simulink model "CompleteModelSimulink"  (R2024a)
settings: Solver=ode45  StartTime=0.0  StopTime=endtime  RelTol=1e-3
values from neighbouring files (symbols this model uses):
  D = 0.069    [CompleteModel.m]
  D_H = 2    [PID_Current.m]    (also in PID_NoCurrent.m = 1)
  D_X = 2    [PID_Current.m]    (also in PID_NoCurrent.m = 1.05)
  D_Y = 2    [PID_Current.m]    (also in PID_NoCurrent.m = 0.8)
  DC =     [DC.mat]
  I_H = 0.1    [PID_Current.m]    (also in PID_NoCurrent.m = 0.01)
  I_X = 0.1    [PID_Current.m]    (also in PID_NoCurrent.m = 0.001)
  I_Y = 0.2    [PID_Current.m]    (also in PID_NoCurrent.m = 0.01)
  InitialPos = [0;0;0]    [CompleteModel.m]
  M_matrix = [2.5 0 0; 0 2.50 0; 0 0 1]    [CompleteModel.m]
  P_H = 2    [PID_Current.m]    (also in PID_NoCurrent.m = 1)
  P_X = 2    [PID_Current.m]    (also in PID_NoCurrent.m = 0.75)
  P_Y = 2    [PID_Current.m]    (also in PID_NoCurrent.m = 1.3)
  Ref = [1;0;0]    [CompleteModel.m]
  SpeedFactor = 0.07    [CompleteModel.m]
  SR =     [SR.mat]
  T_matrix = [0 1 0; 1 0 1; 0.35 -0.065 -0.35]    [CompleteModel.m]
  TauE = [-0.15;0;0]    [CompleteModel.m]
libraries: slpidlib x8
(part 1 of 2)
settings Model: Creator=31620  LastModifiedBy=31620
settings SolverCC: AlgebraicLoopSolver=TrustRegion
settings DebuggingCC: UnconnectedInputMsg=warning  UnconnectedOutputMsg=warning  UnconnectedLineMsg=warning
settings ModelReferenceCC: EnableRefExpFcnMdlSchedulingChecks=on
settings RTWCC: GPUComputeCapability=3.5

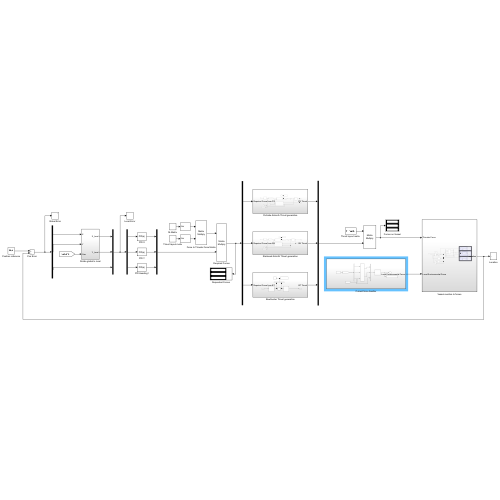
[thumbnail: Simulink's stored preview of the top-level diagram]
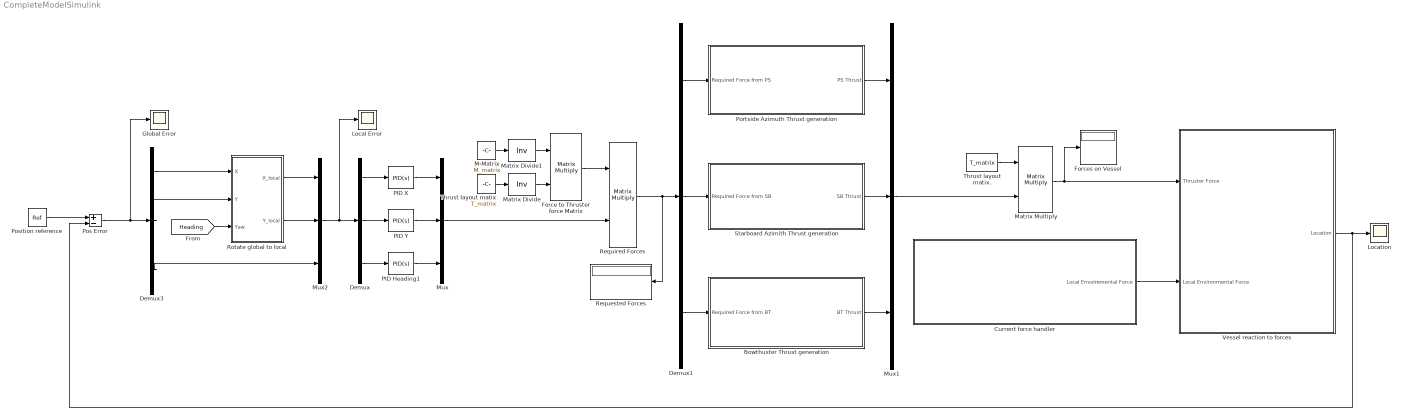
== system CompleteModelSimulink ==
  Bowthuster Thrust generation : Subsystem
  Current force handler : Subsystem
  Demux : Demux  Outputs=3
  Demux1 : Demux  Outputs=3
  Demux3 : Demux  Outputs=3
  Force to Thruster force Matrix : Product  Multiplication=Matrix(*)
  Forces on Vessel : Display
  Global Error : Scope
  Local Error : Scope
  Location : Scope
  M-Matrix : Constant  Value=M_matrix
  Matrix Divide : Product  Inputs=/  Multiplication=Matrix(*)
  Matrix Divide1 : Product  Inputs=/  Multiplication=Matrix(*)
  Matrix Multiply : Product  Multiplication=Matrix(*)
  Mux : Mux  Inputs=3
  Mux1 : Mux  Inputs=3
  Mux2 : Mux  Inputs=3
  PID Heading1 : slpidlib/PID Controller  Controller=PID  Form=Parallel  TimeDomain=Continuous-time  UseExternalTs=off  SampleTime=-1  IntegratorMethod=Forward Euler  FilterMethod=Forward Euler  ControllerParametersSource=internal  P=P_H  I=I_H  UseKiTs=off  D=D_H  UseExternalDerivativeSource=off  N=10000  UseFilter=on  TunerSelectOption=Transfer Function Based (PID Tuner App)  InitialConditionSource=internal  InitialConditionForIntegrator=0  InitialConditionForFilter=0  DifferentiatorICPrevScaledInput=0  ExternalReset=none  TrackingMode=off  Kt=1  LimitOutput=off  SatLimitsSource=internal  UpperSaturationLimit=inf  LowerSaturationLimit=-inf  LinearizeAsGain=on  AntiWindupMode=none  Kb=1  LimitIntegrator=off  UpperIntegratorSaturationLimit=inf  LowerIntegratorSaturationLimit=-inf  POutMin=[]  POutMax=[]  IOutMin=[]  IOutMax=[]  DOutMin=[]  DOutMax=[]  NOutMin=[]  NOutMax=[]  SumOutMin=[]  SumOutMax=[]  SaturationOutMin=[]  SaturationOutMax=[]  PParamMin=[]  PParamMax=[]  IParamMin=[]  IParamMax=[]  DParamMin=[]  DParamMax=[]  NParamMin=[]  NParamMax=[]  KbParamMin=[]  KbParamMax=[]  KtParamMin=[]  KtParamMax=[]  KbOutMin=[]  KbOutMax=[]  KtOutMin=[]  KtOutMax=[]  IntegratorOutMin=[]  IntegratorOutMax=[]  FilterOutMin=[]  FilterOutMax=[]  SumI1OutMin=[]  SumI1OutMax=[]  SumI2OutMin=[]  SumI2OutMax=[]  SumI3OutMin=[]  SumI3OutMax=[]  SumI4OutMin=[]  SumI4OutMax=[]  SumDOutMin=[]  SumDOutMax=[]  DifferentiatorOutMin=[]  DifferentiatorOutMax=[]  FilterDiffOutCoefMin=[]  FilterDiffOutCoefMax=[]  ReciprocalOutMin=[]  ReciprocalOutMax=[]  SumDenOutMin=[]  SumDenOutMax=[]  SumNumOutMin=[]  SumNumOutMax=[]  DivideOutMin=[]  DivideOutMax=[]  UdiffTsProdOutMin=[]  UdiffTsProdOutMax=[]  NTsProdOutMin=[]  NTsProdOutMax=[]  UintegralTsProdOutMin=[]  UintegralTsProdOutMax=[]  UngainTsProdOutMin=[]  UngainTsProdOutMax=[]  ClampingZeroOutDataTypeStr=Inherit: Inherit via back propagation  ClampingZeroOutMin=[]  ClampingZeroOutMax=[]  FilterDenConstantOutDataTypeStr=Inherit: Inherit via back propagation  FilterDenConstantOutMin=[]  FilterDenConstantOutMax=[]  PCopyOutDataTypeStr=Inherit: Inherit via back propagation  PCopyOutMin=[]  PCopyOutMax=[]  NCopyOutDataTypeStr=Inherit: Inherit via back propagation  NCopyOutMin=[]  NCopyOutMax=[]  IntegratorContinuousStateAttributes=''  IntegratorStateMustResolveToSignalObject=off  IntegratorRTWStateStorageClass=Auto  FilterContinuousStateAttributes=''  FilterStateMustResolveToSignalObject=off  FilterRTWStateStorageClass=Auto  ParallelPVariant=InternalParameters  IdealPVariant=Disabled  IVariant=InternalParameters  DVariant=InternalParameters  IntegratorVariant=Continuous  SatVariant=Disabled  AWVariant=Passthrough  PCopyVariant=Disabled  TRVariant=Disabled  FdbkBlocksVariant=Forward  IdealPFdbkVariant=Disabled  SatFdbkVariant=Disabled  DerivativeFilterVariant=ContFilter  NVariant=InternalParameters  NCopyVariant=Disabled  FilterICVariant=InternalICsFilter  IntegratorICVariant=InternalICs  ExternalResetVariant=Disabled  TRSumVariant=Passthrough  SumFdbkVariant=Disabled  SumVariant=Sum_PID  TsampFilterVariant=InternalTs  TsampNgainVariant=Passthrough  TsampIntegralVariant=Disabled_SignalSpec  ExternalSaturationOutDataTypeStr=Inherit: Same as second input  DerivativeSourceVariant=ErrorSignal
  PID X : slpidlib/PID Controller  Controller=PID  Form=Parallel  TimeDomain=Continuous-time  UseExternalTs=off  SampleTime=-1  IntegratorMethod=Forward Euler  FilterMethod=Forward Euler  ControllerParametersSource=internal  P=P_X  I=I_X  UseKiTs=off  D=D_X  UseExternalDerivativeSource=off  N=10000  UseFilter=on  TunerSelectOption=Transfer Function Based (PID Tuner App)  InitialConditionSource=internal  InitialConditionForIntegrator=0  InitialConditionForFilter=0  DifferentiatorICPrevScaledInput=0  ExternalReset=none  TrackingMode=off  Kt=1  LimitOutput=off  SatLimitsSource=internal  UpperSaturationLimit=inf  LowerSaturationLimit=-inf  LinearizeAsGain=on  AntiWindupMode=none  Kb=1  LimitIntegrator=off  UpperIntegratorSaturationLimit=inf  LowerIntegratorSaturationLimit=-inf  POutMin=[]  POutMax=[]  IOutMin=[]  IOutMax=[]  DOutMin=[]  DOutMax=[]  NOutMin=[]  NOutMax=[]  SumOutMin=[]  SumOutMax=[]  SaturationOutMin=[]  SaturationOutMax=[]  PParamMin=[]  PParamMax=[]  IParamMin=[]  IParamMax=[]  DParamMin=[]  DParamMax=[]  NParamMin=[]  NParamMax=[]  KbParamMin=[]  KbParamMax=[]  KtParamMin=[]  KtParamMax=[]  KbOutMin=[]  KbOutMax=[]  KtOutMin=[]  KtOutMax=[]  IntegratorOutMin=[]  IntegratorOutMax=[]  FilterOutMin=[]  FilterOutMax=[]  SumI1OutMin=[]  SumI1OutMax=[]  SumI2OutMin=[]  SumI2OutMax=[]  SumI3OutMin=[]  SumI3OutMax=[]  SumI4OutMin=[]  SumI4OutMax=[]  SumDOutMin=[]  SumDOutMax=[]  DifferentiatorOutMin=[]  DifferentiatorOutMax=[]  FilterDiffOutCoefMin=[]  FilterDiffOutCoefMax=[]  ReciprocalOutMin=[]  ReciprocalOutMax=[]  SumDenOutMin=[]  SumDenOutMax=[]  SumNumOutMin=[]  SumNumOutMax=[]  DivideOutMin=[]  DivideOutMax=[]  UdiffTsProdOutMin=[]  UdiffTsProdOutMax=[]  NTsProdOutMin=[]  NTsProdOutMax=[]  UintegralTsProdOutMin=[]  UintegralTsProdOutMax=[]  UngainTsProdOutMin=[]  UngainTsProdOutMax=[]  ClampingZeroOutDataTypeStr=Inherit: Inherit via back propagation  ClampingZeroOutMin=[]  ClampingZeroOutMax=[]  FilterDenConstantOutDataTypeStr=Inherit: Inherit via back propagation  FilterDenConstantOutMin=[]  FilterDenConstantOutMax=[]  PCopyOutDataTypeStr=Inherit: Inherit via back propagation  PCopyOutMin=[]  PCopyOutMax=[]  NCopyOutDataTypeStr=Inherit: Inherit via back propagation  NCopyOutMin=[]  NCopyOutMax=[]  IntegratorContinuousStateAttributes=''  IntegratorStateMustResolveToSignalObject=off  IntegratorRTWStateStorageClass=Auto  FilterContinuousStateAttributes=''  FilterStateMustResolveToSignalObject=off  FilterRTWStateStorageClass=Auto  ParallelPVariant=InternalParameters  IdealPVariant=Disabled  IVariant=InternalParameters  DVariant=InternalParameters  IntegratorVariant=Continuous  SatVariant=Disabled  AWVariant=Passthrough  PCopyVariant=Disabled  TRVariant=Disabled  FdbkBlocksVariant=Forward  IdealPFdbkVariant=Disabled  SatFdbkVariant=Disabled  DerivativeFilterVariant=ContFilter  NVariant=InternalParameters  NCopyVariant=Disabled  FilterICVariant=InternalICsFilter  IntegratorICVariant=InternalICs  ExternalResetVariant=Disabled  TRSumVariant=Passthrough  SumFdbkVariant=Disabled  SumVariant=Sum_PID  TsampFilterVariant=InternalTs  TsampNgainVariant=Passthrough  TsampIntegralVariant=Disabled_SignalSpec  ExternalSaturationOutDataTypeStr=Inherit: Same as second input  DerivativeSourceVariant=ErrorSignal
  PID Y : slpidlib/PID Controller  Controller=PID  Form=Parallel  TimeDomain=Continuous-time  UseExternalTs=off  SampleTime=-1  IntegratorMethod=Forward Euler  FilterMethod=Forward Euler  ControllerParametersSource=internal  P=P_Y  I=I_Y  UseKiTs=off  D=D_Y  UseExternalDerivativeSource=off  N=10000  UseFilter=on  TunerSelectOption=Transfer Function Based (PID Tuner App)  InitialConditionSource=internal  InitialConditionForIntegrator=0  InitialConditionForFilter=0  DifferentiatorICPrevScaledInput=0  ExternalReset=none  TrackingMode=off  Kt=1  LimitOutput=off  SatLimitsSource=internal  UpperSaturationLimit=inf  LowerSaturationLimit=-inf  LinearizeAsGain=on  AntiWindupMode=none  Kb=1  LimitIntegrator=off  UpperIntegratorSaturationLimit=inf  LowerIntegratorSaturationLimit=-inf  POutMin=[]  POutMax=[]  IOutMin=[]  IOutMax=[]  DOutMin=[]  DOutMax=[]  NOutMin=[]  NOutMax=[]  SumOutMin=[]  SumOutMax=[]  SaturationOutMin=[]  SaturationOutMax=[]  PParamMin=[]  PParamMax=[]  IParamMin=[]  IParamMax=[]  DParamMin=[]  DParamMax=[]  NParamMin=[]  NParamMax=[]  KbParamMin=[]  KbParamMax=[]  KtParamMin=[]  KtParamMax=[]  KbOutMin=[]  KbOutMax=[]  KtOutMin=[]  KtOutMax=[]  IntegratorOutMin=[]  IntegratorOutMax=[]  FilterOutMin=[]  FilterOutMax=[]  SumI1OutMin=[]  SumI1OutMax=[]  SumI2OutMin=[]  SumI2OutMax=[]  SumI3OutMin=[]  SumI3OutMax=[]  SumI4OutMin=[]  SumI4OutMax=[]  SumDOutMin=[]  SumDOutMax=[]  DifferentiatorOutMin=[]  DifferentiatorOutMax=[]  FilterDiffOutCoefMin=[]  FilterDiffOutCoefMax=[]  ReciprocalOutMin=[]  ReciprocalOutMax=[]  SumDenOutMin=[]  SumDenOutMax=[]  SumNumOutMin=[]  SumNumOutMax=[]  DivideOutMin=[]  DivideOutMax=[]  UdiffTsProdOutMin=[]  UdiffTsProdOutMax=[]  NTsProdOutMin=[]  NTsProdOutMax=[]  UintegralTsProdOutMin=[]  UintegralTsProdOutMax=[]  UngainTsProdOutMin=[]  UngainTsProdOutMax=[]  ClampingZeroOutDataTypeStr=Inherit: Inherit via back propagation  ClampingZeroOutMin=[]  ClampingZeroOutMax=[]  FilterDenConstantOutDataTypeStr=Inherit: Inherit via back propagation  FilterDenConstantOutMin=[]  FilterDenConstantOutMax=[]  PCopyOutDataTypeStr=Inherit: Inherit via back propagation  PCopyOutMin=[]  PCopyOutMax=[]  NCopyOutDataTypeStr=Inherit: Inherit via back propagation  NCopyOutMin=[]  NCopyOutMax=[]  IntegratorContinuousStateAttributes=''  IntegratorStateMustResolveToSignalObject=off  IntegratorRTWStateStorageClass=Auto  FilterContinuousStateAttributes=''  FilterStateMustResolveToSignalObject=off  FilterRTWStateStorageClass=Auto  ParallelPVariant=InternalParameters  IdealPVariant=Disabled  IVariant=InternalParameters  DVariant=InternalParameters  IntegratorVariant=Continuous  SatVariant=Disabled  AWVariant=Passthrough  PCopyVariant=Disabled  TRVariant=Disabled  FdbkBlocksVariant=Forward  IdealPFdbkVariant=Disabled  SatFdbkVariant=Disabled  DerivativeFilterVariant=ContFilter  NVariant=InternalParameters  NCopyVariant=Disabled  FilterICVariant=InternalICsFilter  IntegratorICVariant=InternalICs  ExternalResetVariant=Disabled  TRSumVariant=Passthrough  SumFdbkVariant=Disabled  SumVariant=Sum_PID  TsampFilterVariant=InternalTs  TsampNgainVariant=Passthrough  TsampIntegralVariant=Disabled_SignalSpec  ExternalSaturationOutDataTypeStr=Inherit: Same as second input  DerivativeSourceVariant=ErrorSignal
  Portside Azimuth Thrust generation : Subsystem
  Pos Error : Sum  Inputs=+-
  Position reference : Constant  Value=Ref
  Requested Forces : Display
  Required Forces : Product  Multiplication=Matrix(*)
  "Rotate global to local " : Subsystem
  Starboard Azimith Thrust generation : Subsystem
  Thrust layout matix : Constant  Value=T_matrix
  Thrust layout matix. : Constant  Value=T_matrix
  Vessel reaction to forces : Subsystem
  wires:
  Position reference/1 -> Pos Error/1
  Demux/1 -> PID X/1
  Demux/2 -> PID Y/1
  Demux/3 -> PID Heading1/1
  Thrust layout matix/1 -> Matrix Divide/1
  M-Matrix/1 -> Matrix Divide1/1
  Matrix Divide/1 -> Force to Thruster force Matrix/2
  Force to Thruster force Matrix/1 -> Required Forces/1
  Required Forces/1 -> Demux1/1, Requested Forces/1
  Mux1/1 -> Matrix Multiply/2
  Matrix Multiply/1 -> Vessel reaction to forces/1(Thruster Force), Forces on Vessel/1
  Thrust layout matix./1 -> Matrix Multiply/1
  Vessel reaction to forces/1(Location) -> Pos Error/2, Location/1
  Mux/1 -> Required Forces/2
  [Heading] -> "Rotate global to local "/3(Yaw)
  "Rotate global to local "/1(X_local) -> Mux2/1
  "Rotate global to local "/2(Y_local) -> Mux2/2
  Mux2/1 -> Demux/1, Local Error/1
  Demux3/1 -> "Rotate global to local "/1(X)
  Demux3/2 -> "Rotate global to local "/2(Y)
  Pos Error/1 -> Global Error/1, Demux3/1
  Demux3/3 -> Mux2/3
  Matrix Divide1/1 -> Force to Thruster force Matrix/1
  PID Heading1/1 -> Mux/3
  PID Y/1 -> Mux/2
  PID X/1 -> Mux/1
  Demux1/1 -> Portside Azimuth Thrust generation/1(Required Force from PS)
  Portside Azimuth Thrust generation/1(PS Thrust) -> Mux1/1
  Demux1/2 -> Starboard Azimith Thrust generation/1(Required Force from SB)
  Starboard Azimith Thrust generation/1(SB Thrust) -> Mux1/2
  Demux1/3 -> Bowthuster Thrust generation/1(Required Force from BT)
  Bowthuster Thrust generation/1(BT Thrust) -> Mux1/3
  Current force handler/1(Local Envoiremental Force) -> Vessel reaction to forces/2(Local Environmental Force)

== system CompleteModelSimulink/Bowthuster Thrust generation ==
  Required Force from BT : Inport
  "Bow Thruster gain " : Scope
  Force to gain BT : Lookup_n-D  NumberOfTableDimensions=1  BreakpointsForDimension1=[-1.6375;-1.217;-1.0575;-0.92213;-0.78679;-0.47744;-0.16327;-0.005908;0;0.001074;0.059076;0.20892;0.54243;0.73093;1.0016;1.2385;1.3786;1.5526;1.8378]  Table=[-0.64591;-0.54475;-0.49416;-0.44358;-0.39377;-0.2965;-0.19611;-0.098054;0;0.10272;0.20545;0.25214;0.35254;0.40311;0.44825;0.50117;0.55331;0.59922;0.65214]  InternalRulePriority=Speed  RndMeth=Simplest
  Gain to Force BT : Lookup_n-D  NumberOfTableDimensions=1  BreakpointsForDimension1="[-0.645910 -0.544750 -0.49416 -0.443580 -0.39377 -0.2965 -0.19611 -0.098054  0.102720 0.20545 0.25214 0.35254 0.40311 0.448250 0.50117 0.55331 0.59922 0.65214]"  Table="[-1.6375 -1.217 -1.0575 -0.92213 -0.786790 -0.47744 -0.16327 -0.005908  0.001074 0.059076 0.20892 0.542430 0.73093 1.0016 1.2385 1.3786 1.5526 1.8378]"  InternalRulePriority=Speed  RndMeth=Simplest
  Mux6 : Mux  Inputs=2
  Saturation : Saturate  UpperLimit=0.6  LowerLimit=-0.6  ZeroCross=off
  To Workspace : ToWorkspace  VariableName=BowThruster  SaveFormat=Timeseries  SampleTime=-1
  BT Thrust : Outport
  wires:
  Required Force from BT/1 -> Force to gain BT/1
  Gain to Force BT/1 -> BT Thrust/1
  Mux6/1 -> To Workspace/1, "Bow Thruster gain "/1
  Saturation/1 -> Gain to Force BT/1, Mux6/2
  Force to gain BT/1 -> Saturation/1, Mux6/1

== system CompleteModelSimulink/Current force handler ==
  Current Forces : Subsystem
  Demux2 : Demux  Outputs=3
  Envoiremental Force : Constant  Value=TauE
  Gain : Gain  Gain=SpeedFactor
  Mux3 : Mux  Inputs=3
  Rotate global to local : Subsystem
  To Workspace : ToWorkspace  VariableName=LocalEnvoirmentalForce  SaveFormat=Timeseries  SampleTime=-1
  Local Envoiremental Force : Outport
  wires:
  Demux2/2 -> Rotate global to local/2(Y)
  [Heading] -> Rotate global to local/3(Yaw)
  Rotate global to local/2(Y_local) -> Mux3/2
  Demux2/1 -> Rotate global to local/1(X)
  Envoiremental Force/1 -> Gain/1
  Demux2/3 -> Mux3/3
  Gain/1 -> Demux2/1
  Rotate global to local/1(X_local) -> Mux3/1
  Mux3/1 -> Current Forces/1(Snelheid)
  Current Forces/1(D) -> To Workspace/1, Local Envoiremental Force/1

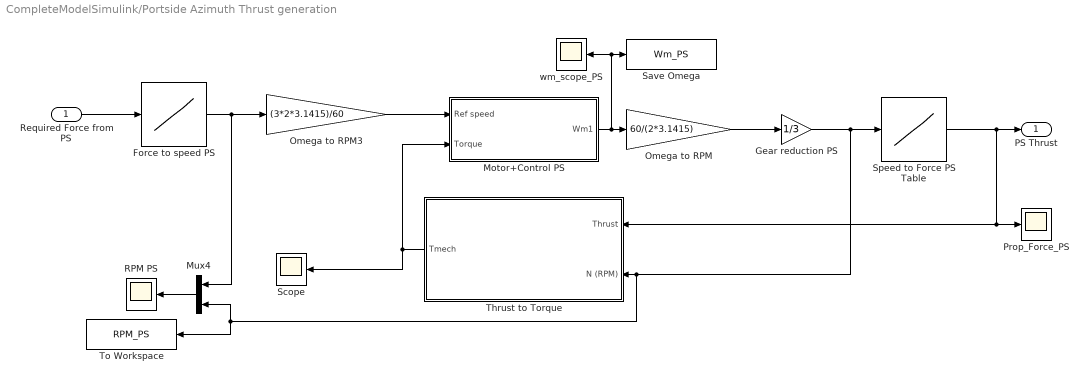
== system CompleteModelSimulink/Portside Azimuth Thrust generation ==
  Required Force from PS : Inport
  Force to speed PS : Lookup_n-D  NumberOfTableDimensions=1  BreakpointsForDimension1=[-2.338 -1.257 -1.059 -0.714 -0.499 -0.329 -0.159 -0.046 0 0.1011 0.2369 0.5481 0.882 1.4196 2.0251 2.789]  BreakpointsForDimension1DataTypeStr=Inherit: Inherit from 'Breakpoint data'  Table=[-998 -801.4 -762.5 -634.8 -563.7 -483.7 -397.1 -339.3 0 299.33 401.52 499.26 620.33 740.28 863.57 1000.2]  TableDataTypeStr=Inherit: Inherit from 'Table data'  RndMeth=Simplest
  Gear reduction PS : Gain  Gain=1/3
  Motor+Control PS : Subsystem
  Mux4 : Mux  Inputs=2
  Omega to RPM : Gain  Gain=60/(2*3.1415)
  Omega to RPM3 : Gain  Gain=(3*2*3.1415)/60
  Prop_Force_PS : Scope
  RPM PS : Scope
  Save Omega : ToWorkspace  VariableName=Wm_PS  SaveFormat=Timeseries  SampleTime=-1
  Scope : Scope
  Speed to Force PS Table : Lookup_n-D  NumberOfTableDimensions=1  BreakpointsForDimension1=[-998 -801.4 -762.5 -634.8 -563.7 -483.7 -397.1 -339.3 0 299.33 401.52 499.26 620.33 740.28 863.57 1000.2]  Table=[-2.338 -1.257 -1.059 -0.714 -0.499 -0.329 -0.159 -0.046 0 0.1011 0.2369 0.5481 0.882 1.4196 2.0251 2.789]  InternalRulePriority=Speed  RndMeth=Simplest
  Thrust to Torque : Subsystem
  To Workspace : ToWorkspace  VariableName=RPM_PS  SaveFormat=Timeseries  SampleTime=-1
  wm_scope_PS : Scope
  PS Thrust : Outport
  wires:
  Mux4/1 -> RPM PS/1
  Speed to Force PS Table/1 -> Thrust to Torque/1(Thrust), Prop_Force_PS/1, PS Thrust/1
  Force to speed PS/1 -> Omega to RPM3/1, Mux4/1
  Motor+Control PS/1(Wm1) -> Omega to RPM/1, wm_scope_PS/1, Save Omega/1
  Omega to RPM/1 -> Gear reduction PS/1
  Gear reduction PS/1 -> Speed to Force PS Table/1, Thrust to Torque/2(N (RPM)), To Workspace/1, Mux4/2
  Omega to RPM3/1 -> Motor+Control PS/1(Ref speed)
  Thrust to Torque/1(Tmech) -> Motor+Control PS/2(Torque), Scope/1
  Required Force from PS/1 -> Force to speed PS/1

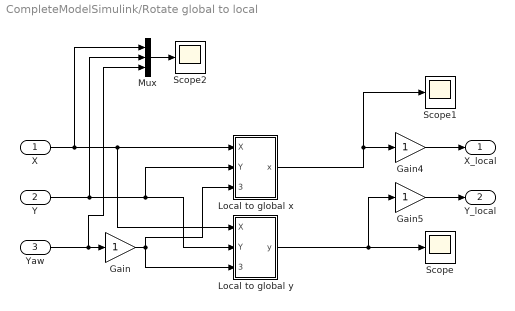
== system CompleteModelSimulink/Rotate global to local  ==
  X : Inport
  Y : Inport  Port=2
  Yaw : Inport  Port=3
  Gain : Gain
  Gain4 : Gain
  Gain5 : Gain
  "Local to global x " : Subsystem
  Local to global y : Subsystem
  Mux : Mux  Inputs=3
  Scope : Scope
  Scope1 : Scope
  Scope2 : Scope
  X_local : Outport  VectorParamsAs1DForOutWhenUnconnected=off
  Y_local : Outport  Port=2  VectorParamsAs1DForOutWhenUnconnected=off
  wires:
  Local to global y/1(y) -> Gain5/1, Scope/1
  Y/1 -> Mux/2, Local to global y/2(Y), "Local to global x "/2(Y)
  "Local to global x "/1(x) -> Scope1/1, Gain4/1
  X/1 -> Mux/1, "Local to global x "/1(X), Local to global y/1(X)
  Yaw/1 -> Mux/3, Gain/1
  Gain/1 -> Local to global y/3(theta), "Local to global x "/3(theta)
  Gain5/1 -> Y_local/1
  Gain4/1 -> X_local/1
  Mux/1 -> Scope2/1

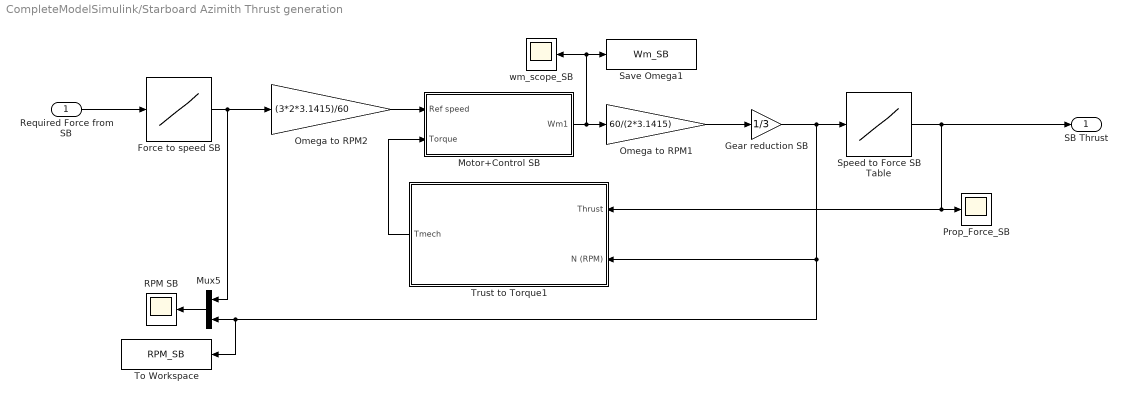
== system CompleteModelSimulink/Starboard Azimith Thrust generation ==
  Required Force from SB : Inport
  Force to speed SB : Lookup_n-D  NumberOfTableDimensions=1  BreakpointsForDimension1=[-1.9091 -1.5672 -1.4695 -1.2659 -0.97286 -0.63908 -0.2483 -0.09362 0 0.052917 0.2483 0.56581 1.1438 1.4613 1.9254 2.5604]  Table=[-1104.9 -1000 -943.82 -900.75 -799.63 -677.9 -501.87 -380.15 0 262.17 466.29 623.6 764.04 863.3 1001.9 1103]  InternalRulePriority=Speed  RndMeth=Simplest
  Gear reduction SB : Gain  Gain=1/3
  Motor+Control SB : Subsystem
  Mux5 : Mux  Inputs=2
  Omega to RPM1 : Gain  Gain=60/(2*3.1415)
  Omega to RPM2 : Gain  Gain=(3*2*3.1415)/60
  Prop_Force_SB : Scope
  RPM SB : Scope
  Save Omega1 : ToWorkspace  VariableName=Wm_SB  SaveFormat=Timeseries  SampleTime=-1
  Speed to Force SB Table : Lookup_n-D  NumberOfTableDimensions=1  BreakpointsForDimension1=[-1104.9 -1000 -943.82 -900.75 -799.63 -677.9 -501.87 -380.15 0 262.17 466.29 623.6 764.04 863.3 1001.9 1103]  Table=[-1.9091 -1.5672 -1.4695 -1.2659 -0.97286 -0.63908 -0.2483 -0.09362 0 0.052917 0.2483 0.56581 1.1438 1.4613 1.9254 2.5604]  InternalRulePriority=Speed  RndMeth=Simplest
  To Workspace : ToWorkspace  VariableName=RPM_SB  SaveFormat=Timeseries  SampleTime=-1
  Trust to Torque1 : Subsystem
  wm_scope_SB : Scope
  SB Thrust : Outport
  wires:
  Motor+Control SB/1(Wm1) -> wm_scope_SB/1, Save Omega1/1, Omega to RPM1/1
  Required Force from SB/1 -> Force to speed SB/1
  Omega to RPM2/1 -> Motor+Control SB/1(Ref speed)
  Gear reduction SB/1 -> Speed to Force SB Table/1, Mux5/2, To Workspace/1, Trust to Torque1/2(N (RPM))
  Omega to RPM1/1 -> Gear reduction SB/1
  Speed to Force SB Table/1 -> Trust to Torque1/1(Thrust), Prop_Force_SB/1, SB Thrust/1
  Force to speed SB/1 -> Mux5/1, Omega to RPM2/1
  Trust to Torque1/1(Tmech) -> Motor+Control SB/2(Torque)
  Mux5/1 -> RPM SB/1

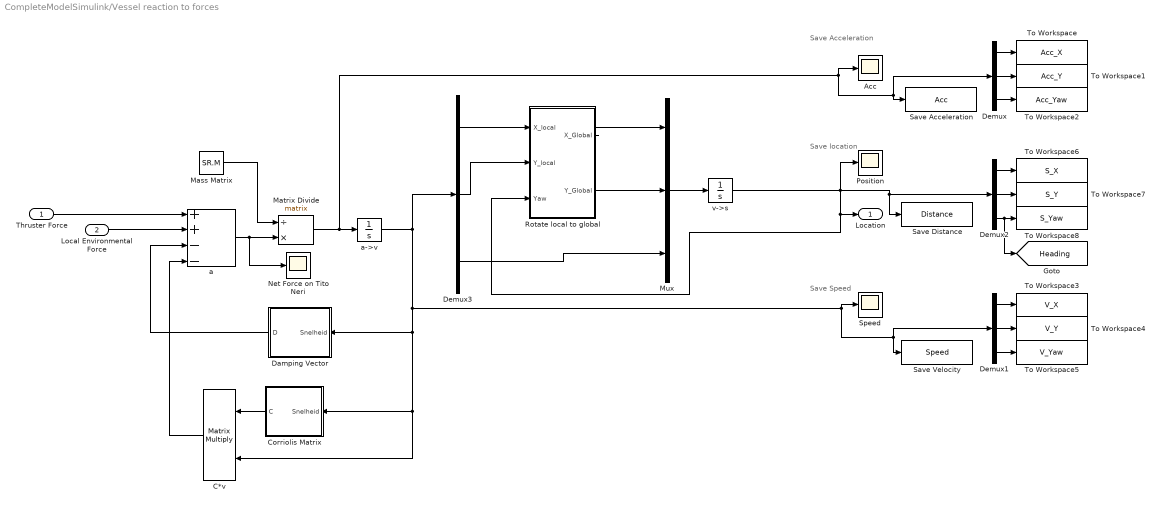
== system CompleteModelSimulink/Vessel reaction to forces ==
  note: Save location
  note: Save Speed
  note: Save Acceleration
  Thruster Force : Inport
  Local Environmental Force : Inport  Port=2
  Acc : Scope
  C*v : Product  Multiplication=Matrix(*)
  Corriolis Matrix : Subsystem
  Damping Vector : Subsystem
  Demux{,1..3} (4 alike) : Demux  Outputs=3
  Mass Matrix : Constant  Value=SR.M
  Matrix Divide : Product  Inputs=/*  Multiplication=Matrix(*)
  Mux : Mux  Inputs=3
  Net Force on Tito Neri : Scope
  Position : Scope
  "Rotate local to global " : Subsystem
  Save Acceleration : ToWorkspace  VariableName=Acc  SampleTime=-1
      settings: Decimation=2  Save2DSignal=2-D array (concatenate along first dimension)
  Save Distance : ToWorkspace  VariableName=Distance  SampleTime=-1
      settings: Save2DSignal=2-D array (concatenate along first dimension)
  Save Velocity : ToWorkspace  VariableName=Speed  SampleTime=-1
      settings: Save2DSignal=2-D array (concatenate along first dimension)
  Speed : Scope
  To Workspace : ToWorkspace  VariableName=Acc_X  SaveFormat=Timeseries  SampleTime=-1
  To Workspace1 : ToWorkspace  VariableName=Acc_Y  SaveFormat=Timeseries  SampleTime=-1
  To Workspace2 : ToWorkspace  VariableName=Acc_Yaw  SaveFormat=Timeseries  SampleTime=-1
  To Workspace3 : ToWorkspace  VariableName=V_X  SaveFormat=Timeseries  SampleTime=-1
  To Workspace4 : ToWorkspace  VariableName=V_Y  SaveFormat=Timeseries  SampleTime=-1
  To Workspace5 : ToWorkspace  VariableName=V_Yaw  SaveFormat=Timeseries  SampleTime=-1
  To Workspace6 : ToWorkspace  VariableName=S_X  SaveFormat=Timeseries  SampleTime=-1
  To Workspace7 : ToWorkspace  VariableName=S_Y  SaveFormat=Timeseries  SampleTime=-1
  To Workspace8 : ToWorkspace  VariableName=S_Yaw  SaveFormat=Timeseries  SampleTime=-1
  a : Sum  Inputs=++--
  a->v : Integrator  InitialCondition=[0;0;0]
  v->s : Integrator  InitialCondition=InitialPos
  Location : Outport
  tag scope: Heading=global
  wires:
  a/1 -> Net Force on Tito Neri/1, Matrix Divide/2
  Corriolis Matrix/1(C) -> C*v/1
  Mass Matrix/1 -> Matrix Divide/1
  Damping Vector/1(D) -> a/3
  C*v/1 -> a/4
  Matrix Divide/1 -> a->v/1, Save Acceleration/1, Demux/1, Acc/1
  Thruster Force/1 -> a/1
  a->v/1 -> Demux3/1, Corriolis Matrix/1(Snelheid), C*v/2, Damping Vector/1(Snelheid), Speed/1, Demux1/1, Save Velocity/1
  Demux/1 -> To Workspace/1
  Demux/2 -> To Workspace1/1
  Demux/3 -> To Workspace2/1
  Demux1/1 -> To Workspace3/1
  Demux1/2 -> To Workspace4/1
  Demux1/3 -> To Workspace5/1
  Demux2/1 -> To Workspace6/1
  Demux2/2 -> To Workspace7/1
  Demux2/3 -> [Heading], To Workspace8/1
  Demux3/1 -> "Rotate local to global "/1(X_local)
  Demux3/2 -> "Rotate local to global "/2(Y_local)
  "Rotate local to global "/1(X_Global) -> Mux/1
  "Rotate local to global "/2(Y_Global) -> Mux/2
  Mux/1 -> v->s/1
  v->s/1 -> Location/1, "Rotate local to global "/3(Yaw), Demux2/1, Save Distance/1, Position/1
  Local Environmental Force/1 -> a/2
  Demux3/3 -> Mux/3

== system CompleteModelSimulink/Current force handler/Current Forces ==
  Snelheid : Inport
  Damping : MATLAB Function  TreatAsAtomicUnit=on
  Length : Constant  Value=SR.L
  Xdrag_coef : Constant  Value=SR.Xdrag_coef
  Yaw_coef : Constant  Value=SR.Yaw_coef
  Ydrag_coef : Constant  Value=SR.Ydrag_coef
  D : Outport
  wires:
  Length/1 -> Damping/5(L)
  Ydrag_coef/1 -> Damping/3(Y)
  Yaw_coef/1 -> Damping/4(Yaw)
  Xdrag_coef/1 -> Damping/2(X)
  Snelheid/1 -> Damping/1(uvr)
  Damping/1(D) -> D/1

== system CompleteModelSimulink/Current force handler/Rotate global to local ==
  X : Inport
  Y : Inport  Port=2
  Yaw : Inport  Port=3
  Gain : Gain
  Gain4 : Gain
  Gain5 : Gain
  "Local to global x " : Subsystem
  Local to global y : Subsystem
  X_local : Outport  VectorParamsAs1DForOutWhenUnconnected=off
  Y_local : Outport  Port=2  VectorParamsAs1DForOutWhenUnconnected=off
  wires:
  Local to global y/1(y) -> Gain5/1
  Y/1 -> Local to global y/2(Y), "Local to global x "/2(Y)
  "Local to global x "/1(x) -> Gain4/1
  X/1 -> Local to global y/1(X), "Local to global x "/1(X)
  Yaw/1 -> Gain/1
  Gain/1 -> Local to global y/3(theta), "Local to global x "/3(theta)
  Gain5/1 -> Y_local/1
  Gain4/1 -> X_local/1

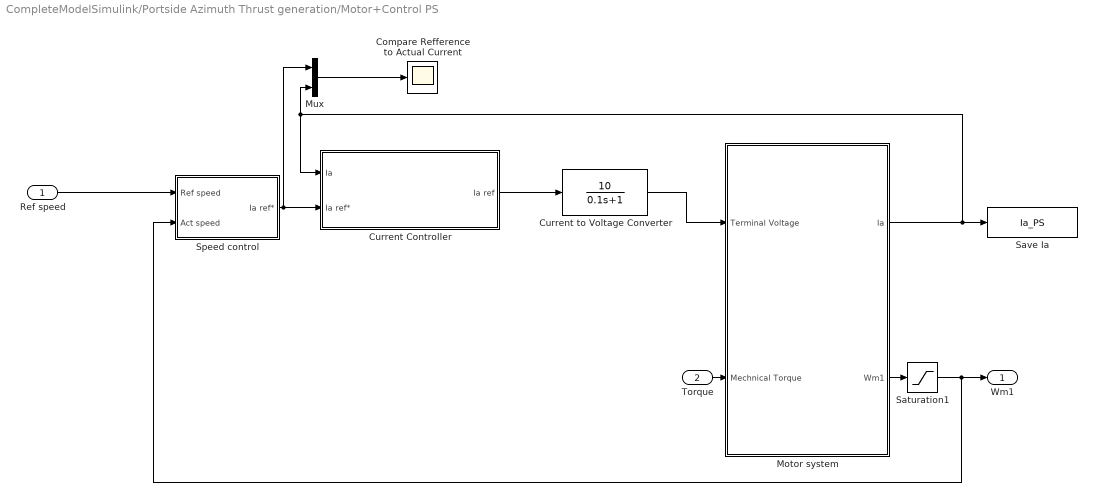
== system CompleteModelSimulink/Portside Azimuth Thrust generation/Motor+Control PS ==
  Ref speed : Inport
  Torque : Inport  Port=2
  Compare Refference to Actual Current : Scope
  Current Controller : Subsystem
  Current to Voltage Converter : TransferFcn  Numerator=[10]  Denominator=[0.1 1]
  Motor system : Subsystem
  Mux : Mux  Inputs=2
  Saturation1 : Saturate  UpperLimit=315  LowerLimit=-315
  Save Ia : ToWorkspace  VariableName=Ia_PS  SaveFormat=Timeseries  SampleTime=-1
  Speed control : Subsystem
  Wm1 : Outport
  wires:
  Motor system/1(Ia) -> Mux/2, Current Controller/1(Ia), Save Ia/1
  Current to Voltage Converter/1 -> Motor system/1(Terminal Voltage)
  Current Controller/1(Ia ref) -> Current to Voltage Converter/1
  Speed control/1(Ia ref*) -> Mux/1, Current Controller/2(Ia ref*)
  Ref speed/1 -> Speed control/1(Ref speed)
  Saturation1/1 -> Speed control/2(Act speed), Wm1/1
  Motor system/2(Wm1) -> Saturation1/1
  Torque/1 -> Motor system/2(Mechnical Torque)
  Mux/1 -> Compare Refference to Actual Current/1

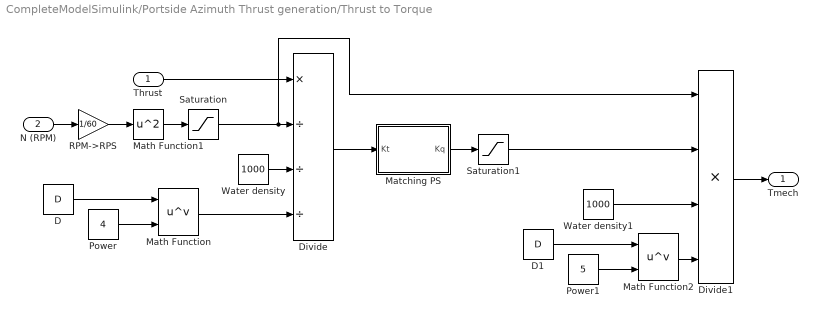
== system CompleteModelSimulink/Portside Azimuth Thrust generation/Thrust to Torque ==
  Thrust : Inport
  N (RPM) : Inport  Port=2
  D : Constant  Value=D
  D1 : Constant  Value=D
  Divide : Product  Inputs=*///
  Divide1 : Product  Inputs=****
  Matching PS : MATLAB Function  TreatAsAtomicUnit=on
  Math Function : Math  Operator=pow  OutputSignalType=real
  Math Function1 : Math  Operator=square
  Math Function2 : Math  Operator=pow  OutputSignalType=real
  Power : Constant  Value=4
  Power1 : Constant  Value=5
  RPM->RPS : Gain  Gain=1/60
  Saturation : Saturate  UpperLimit=10000  LowerLimit=0.1
  Saturation1 : Saturate  UpperLimit=0.051282051  LowerLimit=0
  Water density : Constant  Value=1000
  Water density1 : Constant  Value=1000
  Tmech : Outport
  wires:
  Thrust/1 -> Divide/1
  Divide1/1 -> Tmech/1
  Power/1 -> Math Function/2
  D/1 -> Math Function/1
  N (RPM)/1 -> RPM->RPS/1
  RPM->RPS/1 -> Math Function1/1
  Math Function1/1 -> Saturation/1
  Water density/1 -> Divide/3
  Math Function/1 -> Divide/4
  Divide/1 -> Matching PS/1(Kt)
  D1/1 -> Math Function2/1
  Math Function2/1 -> Divide1/4
  Power1/1 -> Math Function2/2
  Matching PS/1(Kq) -> Saturation1/1
  Water density1/1 -> Divide1/3
  Saturation/1 -> Divide1/1, Divide/2
  Saturation1/1 -> Divide1/2

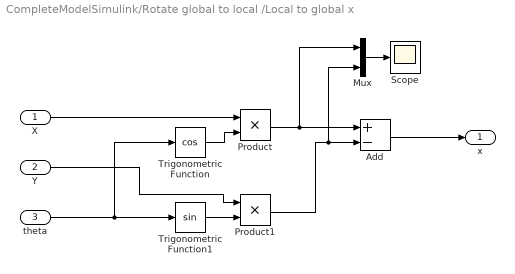
== system CompleteModelSimulink/Rotate global to local /Local to global x  ==
  X : Inport
  Y : Inport  Port=2
  theta : Inport  Port=3
  Add : Sum  Inputs=+-
  Mux : Mux  Inputs=2
  Product : Product
  Product1 : Product
  Scope : Scope
  Trigonometric Function : Trigonometry  Operator=cos
  Trigonometric Function1 : Trigonometry
  x : Outport  VectorParamsAs1DForOutWhenUnconnected=off
  wires:
  Add/1 -> x/1
  Product1/1 -> Mux/2, Add/2
  Product/1 -> Mux/1, Add/1
  Y/1 -> Product1/1
  X/1 -> Product/1
  theta/1 -> Trigonometric Function1/1, Trigonometric Function/1
  Trigonometric Function1/1 -> Product1/2
  Trigonometric Function/1 -> Product/2
  Mux/1 -> Scope/1

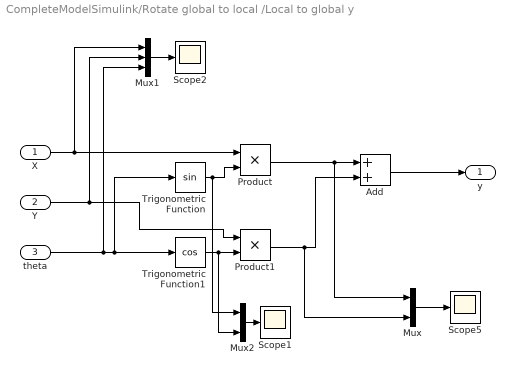
== system CompleteModelSimulink/Rotate global to local /Local to global y ==
  X : Inport
  Y : Inport  Port=2
  theta : Inport  Port=3
  Add : Sum
  Mux : Mux  Inputs=2
  Mux1 : Mux  Inputs=3
  Mux2 : Mux  Inputs=2
  Product : Product
  Product1 : Product
  Scope1 : Scope
  Scope2 : Scope
  Scope5 : Scope
  Trigonometric Function : Trigonometry  OutputSignalType=real
  Trigonometric Function1 : Trigonometry  Operator=cos  OutputSignalType=real
  y : Outport  VectorParamsAs1DForOutWhenUnconnected=off
  wires:
  Add/1 -> y/1
  Product/1 -> Add/1, Mux/1
  Product1/1 -> Add/2, Mux/2
  Mux/1 -> Scope5/1
  X/1 -> Mux1/1, Product/1
  Mux1/1 -> Scope2/1
  theta/1 -> Mux1/3, Trigonometric Function1/1, Trigonometric Function/1
  Y/1 -> Mux1/2, Product1/1
  Trigonometric Function1/1 -> Mux2/2, Product1/2
  Trigonometric Function/1 -> Product/2, Mux2/1
  Mux2/1 -> Scope1/1

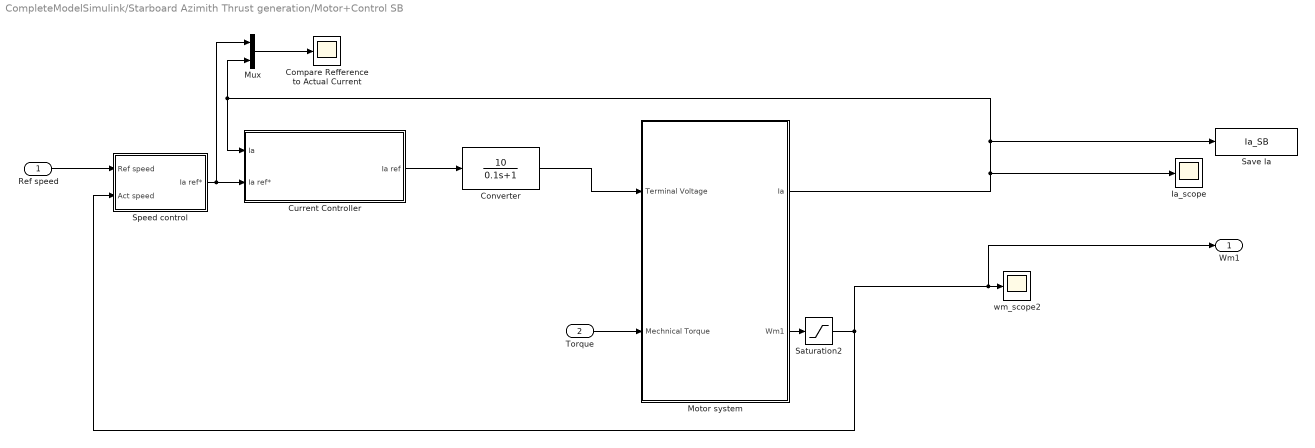
== system CompleteModelSimulink/Starboard Azimith Thrust generation/Motor+Control SB ==
  Ref speed : Inport
  Torque : Inport  Port=2
  Compare Refference to Actual Current : Scope
  Converter : TransferFcn  Numerator=[10]  Denominator=[0.1 1]
  Current Controller : Subsystem
  Ia_scope : Scope
  Motor system : Subsystem
  Mux : Mux  Inputs=2
  Saturation2 : Saturate  UpperLimit=315  LowerLimit=-315
  Save Ia : ToWorkspace  VariableName=Ia_SB  SaveFormat=Timeseries  SampleTime=-1
  Speed control : Subsystem
  wm_scope2 : Scope
  Wm1 : Outport
  wires:
  Converter/1 -> Motor system/1(Terminal Voltage)
  Current Controller/1(Ia ref) -> Converter/1
  Ref speed/1 -> Speed control/1(Ref speed)
  Saturation2/1 -> Speed control/2(Act speed), Wm1/1, wm_scope2/1
  Motor system/2(Wm1) -> Saturation2/1
  Torque/1 -> Motor system/2(Mechnical Torque)
  Mux/1 -> Compare Refference to Actual Current/1
  Speed control/1(Ia ref*) -> Mux/1, Current Controller/2(Ia ref*)
  Motor system/1(Ia) -> Save Ia/1, Mux/2, Current Controller/1(Ia), Ia_scope/1

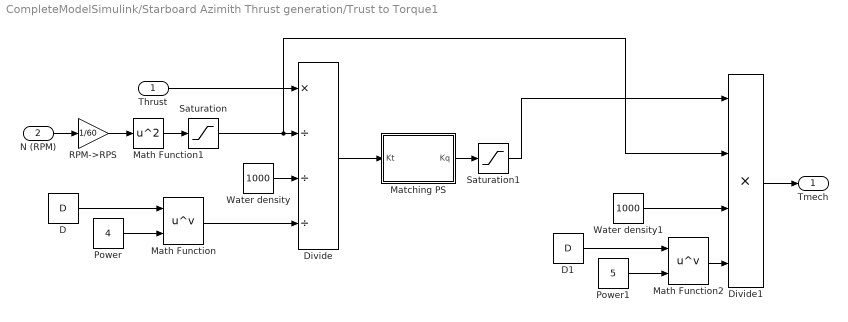
== system CompleteModelSimulink/Starboard Azimith Thrust generation/Trust to Torque1 ==
  Thrust : Inport
  N (RPM) : Inport  Port=2
  D : Constant  Value=D
  D1 : Constant  Value=D
  Divide : Product  Inputs=*///
  Divide1 : Product  Inputs=****
  Matching PS : MATLAB Function  TreatAsAtomicUnit=on
  Math Function : Math  Operator=pow  OutputSignalType=real
  Math Function1 : Math  Operator=square
  Math Function2 : Math  Operator=pow  OutputSignalType=real
  Power : Constant  Value=4
  Power1 : Constant  Value=5
  RPM->RPS : Gain  Gain=1/60
  Saturation : Saturate  UpperLimit=10000  LowerLimit=0.1
  Saturation1 : Saturate  UpperLimit=0.051282051  LowerLimit=0
  Water density : Constant  Value=1000
  Water density1 : Constant  Value=1000
  Tmech : Outport
  wires:
  Thrust/1 -> Divide/1
  Divide1/1 -> Tmech/1
  Power/1 -> Math Function/2
  D/1 -> Math Function/1
  N (RPM)/1 -> RPM->RPS/1
  RPM->RPS/1 -> Math Function1/1
  Math Function1/1 -> Saturation/1
  Water density/1 -> Divide/3
  Math Function/1 -> Divide/4
  Divide/1 -> Matching PS/1(Kt)
  D1/1 -> Math Function2/1
  Math Function2/1 -> Divide1/4
  Power1/1 -> Math Function2/2
  Matching PS/1(Kq) -> Saturation1/1
  Water density1/1 -> Divide1/3
  Saturation/1 -> Divide1/2, Divide/2
  Saturation1/1 -> Divide1/1

== system CompleteModelSimulink/Vessel reaction to forces/Corriolis Matrix ==
  Snelheid : Inport
  MATLAB Function1 : MATLAB Function  TreatAsAtomicUnit=on
  Mass : Constant  Value=SR.m
  Scope : Scope
  Xudot : Constant  Value=SR.Xudot
  Yvdot : Constant  Value=SR.Yvdot
  C : Outport
  wires:
  Yvdot/1 -> MATLAB Function1/3(Yvdot)
  MATLAB Function1/1(C) -> C/1
  Xudot/1 -> MATLAB Function1/2(Xudot)
  Mass/1 -> MATLAB Function1/4(m)
  Snelheid/1 -> Scope/1, MATLAB Function1/1(uv)

== system CompleteModelSimulink/Vessel reaction to forces/Damping Vector ==
  Snelheid : Inport
  Damping : MATLAB Function  TreatAsAtomicUnit=on
  Length : Constant  Value=SR.L
  Xdrag_coef : Constant  Value=SR.Xdrag_coef
  Yaw_coef : Constant  Value=SR.Yaw_coef
  Ydrag_coef : Constant  Value=SR.Ydrag_coef
  D : Outport
  wires:
  Length/1 -> Damping/5(L)
  Ydrag_coef/1 -> Damping/3(Y)
  Yaw_coef/1 -> Damping/4(Yaw)
  Xdrag_coef/1 -> Damping/2(X)
  Snelheid/1 -> Damping/1(uvr)
  Damping/1(D) -> D/1

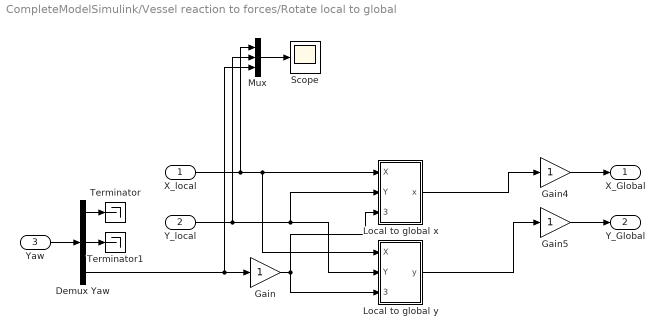
== system CompleteModelSimulink/Vessel reaction to forces/Rotate local to global  ==
  X_local : Inport
  Y_local : Inport  Port=2
  Yaw : Inport  Port=3
  Demux Yaw : Demux  Outputs=3
  Gain : Gain
  Gain4 : Gain
  Gain5 : Gain
  "Local to global x " : Subsystem
  Local to global y : Subsystem
  Mux : Mux  Inputs=3
  Scope : Scope
  Terminator : Terminator
  Terminator1 : Terminator
  X_Global : Outport  VectorParamsAs1DForOutWhenUnconnected=off
  Y_Global : Outport  Port=2  VectorParamsAs1DForOutWhenUnconnected=off
  wires:
  Local to global y/1(y) -> Gain5/1
  "Local to global x "/1(x) -> Gain4/1
  X_local/1 -> Mux/1, Local to global y/1(X), "Local to global x "/1(X)
  Gain/1 -> Local to global y/3(theta), "Local to global x "/3(theta)
  Gain5/1 -> Y_Global/1
  Gain4/1 -> X_Global/1
  Demux Yaw/1 -> Terminator/1
  Yaw/1 -> Demux Yaw/1
  Demux Yaw/2 -> Terminator1/1
  Demux Yaw/3 -> Mux/3, Gain/1
  Mux/1 -> Scope/1
  Y_local/1 -> Mux/2, Local to global y/2(Y), "Local to global x "/2(Y)

== system CompleteModelSimulink/Current force handler/Rotate global to local/Local to global x  ==
  X : Inport
  Y : Inport  Port=2
  theta : Inport  Port=3
  Add : Sum  Inputs=+-
  Product : Product
  Product1 : Product
  Trigonometric Function : Trigonometry  Operator=cos
  Trigonometric Function1 : Trigonometry
  x : Outport  VectorParamsAs1DForOutWhenUnconnected=off
  wires:
  Add/1 -> x/1
  Product1/1 -> Add/2
  Product/1 -> Add/1
  Y/1 -> Product1/1
  X/1 -> Product/1
  theta/1 -> Trigonometric Function1/1, Trigonometric Function/1
  Trigonometric Function1/1 -> Product1/2
  Trigonometric Function/1 -> Product/2

== system CompleteModelSimulink/Current force handler/Rotate global to local/Local to global y ==
  X : Inport
  Y : Inport  Port=2
  theta : Inport  Port=3
  Add : Sum
  Product : Product
  Product1 : Product
  Trigonometric Function : Trigonometry
  Trigonometric Function1 : Trigonometry  Operator=cos
  y : Outport  VectorParamsAs1DForOutWhenUnconnected=off
  wires:
  Add/1 -> y/1
  Product1/1 -> Add/2
  Product/1 -> Add/1
  Y/1 -> Product1/1
  X/1 -> Product/1
  theta/1 -> Trigonometric Function1/1, Trigonometric Function/1
  Trigonometric Function1/1 -> Product1/2
  Trigonometric Function/1 -> Product/2

== system CompleteModelSimulink/Portside Azimuth Thrust generation/Motor+Control PS/Current Controller ==
  Ia : Inport
  Ia ref* : Inport  Port=2
  Constant : Constant  Value=DC.Irated
  Error : Sum  Inputs=|+-
  Normalise : Product  Inputs=*/
  PID Controller : slpidlib/PID Controller  Controller=PID  Form=Ideal  TimeDomain=Continuous-time  UseExternalTs=off  SampleTime=-1  IntegratorMethod=Forward Euler  FilterMethod=Forward Euler  ControllerParametersSource=internal  P=7.2353580328522  I=2.78600690342995  UseKiTs=off  D=0.0824758010540437  UseExternalDerivativeSource=off  N=135.726193036092  UseFilter=on  TunerSelectOption=Transfer Function Based (PID Tuner App)  InitialConditionSource=internal  InitialConditionForIntegrator=0  InitialConditionForFilter=0  DifferentiatorICPrevScaledInput=0  ExternalReset=none  TrackingMode=off  Kt=1  LimitOutput=on  SatLimitsSource=internal  UpperSaturationLimit=1.2*DC.Irated  LowerSaturationLimit=-0.5*DC.Irated  LinearizeAsGain=on  AntiWindupMode=back-calculation  Kb=14  LimitIntegrator=off  UpperIntegratorSaturationLimit=inf  LowerIntegratorSaturationLimit=-inf  POutMin=[]  POutMax=[]  IOutMin=[]  IOutMax=[]  DOutMin=[]  DOutMax=[]  NOutMin=[]  NOutMax=[]  SumOutMin=[]  SumOutMax=[]  SaturationOutMin=[]  SaturationOutMax=[]  PParamMin=[]  PParamMax=[]  IParamMin=[]  IParamMax=[]  DParamMin=[]  DParamMax=[]  NParamMin=[]  NParamMax=[]  KbParamMin=[]  KbParamMax=[]  KtParamMin=[]  KtParamMax=[]  KbOutMin=[]  KbOutMax=[]  KtOutMin=[]  KtOutMax=[]  IntegratorOutMin=[]  IntegratorOutMax=[]  FilterOutMin=[]  FilterOutMax=[]  SumI1OutMin=[]  SumI1OutMax=[]  SumI2OutMin=[]  SumI2OutMax=[]  SumI3OutMin=[]  SumI3OutMax=[]  SumI4OutMin=[]  SumI4OutMax=[]  SumDOutMin=[]  SumDOutMax=[]  DifferentiatorOutMin=[]  DifferentiatorOutMax=[]  FilterDiffOutCoefMin=[]  FilterDiffOutCoefMax=[]  ReciprocalOutMin=[]  ReciprocalOutMax=[]  SumDenOutMin=[]  SumDenOutMax=[]  SumNumOutMin=[]  SumNumOutMax=[]  DivideOutMin=[]  DivideOutMax=[]  UdiffTsProdOutMin=[]  UdiffTsProdOutMax=[]  NTsProdOutMin=[]  NTsProdOutMax=[]  UintegralTsProdOutMin=[]  UintegralTsProdOutMax=[]  UngainTsProdOutMin=[]  UngainTsProdOutMax=[]  ClampingZeroOutDataTypeStr=Inherit: Inherit via back propagation  ClampingZeroOutMin=[]  ClampingZeroOutMax=[]  FilterDenConstantOutDataTypeStr=Inherit: Inherit via back propagation  FilterDenConstantOutMin=[]  FilterDenConstantOutMax=[]  PCopyOutDataTypeStr=Inherit: Inherit via back propagation  PCopyOutMin=[]  PCopyOutMax=[]  NCopyOutDataTypeStr=Inherit: Inherit via back propagation  NCopyOutMin=[]  NCopyOutMax=[]  IntegratorContinuousStateAttributes=''  IntegratorStateMustResolveToSignalObject=off  IntegratorRTWStateStorageClass=Auto  FilterContinuousStateAttributes=''  FilterStateMustResolveToSignalObject=off  FilterRTWStateStorageClass=Auto  ParallelPVariant=Passthrough  IdealPVariant=InternalParameters  IVariant=InternalParameters  DVariant=InternalParameters  IntegratorVariant=Continuous  SatVariant=Enabled  AWVariant=BackCalculation  PCopyVariant=Disabled  TRVariant=Disabled  FdbkBlocksVariant=Forward  IdealPFdbkVariant=Disabled  SatFdbkVariant=Disabled  DerivativeFilterVariant=ContFilter  NVariant=InternalParameters  NCopyVariant=Disabled  FilterICVariant=InternalICsFilter  IntegratorICVariant=InternalICs  ExternalResetVariant=Disabled  TRSumVariant=Passthrough  SumFdbkVariant=Disabled  SumVariant=Sum_PID  TsampFilterVariant=InternalTs  TsampNgainVariant=Passthrough  TsampIntegralVariant=Disabled_SignalSpec  ExternalSaturationOutDataTypeStr=Inherit: Same as second input  DerivativeSourceVariant=ErrorSignal
  Ia ref : Outport
  wires:
  Error/1 -> Normalise/1
  Normalise/1 -> PID Controller/1
  Ia/1 -> Error/2
  PID Controller/1 -> Ia ref/1
  Ia ref*/1 -> Error/1
  Constant/1 -> Normalise/2

== system CompleteModelSimulink/Portside Azimuth Thrust generation/Motor+Control PS/Motor system ==
  Terminal Voltage : Inport
  Mechnical Torque : Inport  Port=2
  Electrical Equation : Subsystem
  Mechnical Equation : Subsystem
  Ia : Outport
  Wm1 : Outport  Port=2
  wires:
  Electrical Equation/1(Ia) -> Ia/1, Mechnical Equation/1(Ia)
  Mechnical Torque/1 -> Mechnical Equation/2(Mechnical Torque)
  Terminal Voltage/1 -> Electrical Equation/1(Terminal Voltage)
  Mechnical Equation/1(Wm) -> Wm1/1, Electrical Equation/2(Wm)

== system CompleteModelSimulink/Portside Azimuth Thrust generation/Motor+Control PS/Speed control ==
  Ref speed : Inport
  Act speed : Inport  Port=2
  Constant : Constant  Value=DC.Omegarated
  Divide : Product  Inputs=/*
  PID Controller2 : slpidlib/PID Controller  Controller=PID  Form=Ideal  TimeDomain=Continuous-time  UseExternalTs=off  SampleTime=-1  IntegratorMethod=Forward Euler  FilterMethod=Forward Euler  ControllerParametersSource=internal  P=301.958567368747  I=2.49617195964231  UseKiTs=off  D=0.0354093832005891  UseExternalDerivativeSource=off  N=1725.20945072566  UseFilter=on  TunerSelectOption=Transfer Function Based (PID Tuner App)  InitialConditionSource=internal  InitialConditionForIntegrator=0  InitialConditionForFilter=0  DifferentiatorICPrevScaledInput=0  ExternalReset=none  TrackingMode=off  Kt=1  LimitOutput=on  SatLimitsSource=internal  UpperSaturationLimit=1.2*DC.Irated  LowerSaturationLimit=-0.5*DC.Irated  LinearizeAsGain=off  AntiWindupMode=back-calculation  Kb=14  LimitIntegrator=off  UpperIntegratorSaturationLimit=inf  LowerIntegratorSaturationLimit=-inf  POutMin=[]  POutMax=[]  IOutMin=[]  IOutMax=[]  DOutMin=[]  DOutMax=[]  NOutMin=[]  NOutMax=[]  SumOutMin=[]  SumOutMax=[]  SaturationOutMin=[]  SaturationOutMax=[]  PParamMin=[]  PParamMax=[]  IParamMin=[]  IParamMax=[]  DParamMin=[]  DParamMax=[]  NParamMin=[]  NParamMax=[]  KbParamMin=[]  KbParamMax=[]  KtParamMin=[]  KtParamMax=[]  KbOutMin=[]  KbOutMax=[]  KtOutMin=[]  KtOutMax=[]  IntegratorOutMin=[]  IntegratorOutMax=[]  FilterOutMin=[]  FilterOutMax=[]  SumI1OutMin=[]  SumI1OutMax=[]  SumI2OutMin=[]  SumI2OutMax=[]  SumI3OutMin=[]  SumI3OutMax=[]  SumI4OutMin=[]  SumI4OutMax=[]  SumDOutMin=[]  SumDOutMax=[]  DifferentiatorOutMin=[]  DifferentiatorOutMax=[]  FilterDiffOutCoefMin=[]  FilterDiffOutCoefMax=[]  ReciprocalOutMin=[]  ReciprocalOutMax=[]  SumDenOutMin=[]  SumDenOutMax=[]  SumNumOutMin=[]  SumNumOutMax=[]  DivideOutMin=[]  DivideOutMax=[]  UdiffTsProdOutMin=[]  UdiffTsProdOutMax=[]  NTsProdOutMin=[]  NTsProdOutMax=[]  UintegralTsProdOutMin=[]  UintegralTsProdOutMax=[]  UngainTsProdOutMin=[]  UngainTsProdOutMax=[]  ClampingZeroOutDataTypeStr=Inherit: Inherit via back propagation  ClampingZeroOutMin=[]  ClampingZeroOutMax=[]  FilterDenConstantOutDataTypeStr=Inherit: Inherit via back propagation  FilterDenConstantOutMin=[]  FilterDenConstantOutMax=[]  PCopyOutDataTypeStr=Inherit: Inherit via back propagation  PCopyOutMin=[]  PCopyOutMax=[]  NCopyOutDataTypeStr=Inherit: Inherit via back propagation  NCopyOutMin=[]  NCopyOutMax=[]  IntegratorContinuousStateAttributes=''  IntegratorStateMustResolveToSignalObject=off  IntegratorRTWStateStorageClass=Auto  FilterContinuousStateAttributes=''  FilterStateMustResolveToSignalObject=off  FilterRTWStateStorageClass=Auto  ParallelPVariant=Passthrough  IdealPVariant=InternalParameters  IVariant=InternalParameters  DVariant=InternalParameters  IntegratorVariant=Continuous  SatVariant=Enabled  AWVariant=BackCalculation  PCopyVariant=Disabled  TRVariant=Disabled  FdbkBlocksVariant=Forward  IdealPFdbkVariant=Disabled  SatFdbkVariant=Disabled  DerivativeFilterVariant=ContFilter  NVariant=InternalParameters  NCopyVariant=Disabled  FilterICVariant=InternalICsFilter  IntegratorICVariant=InternalICs  ExternalResetVariant=Disabled  TRSumVariant=Passthrough  SumFdbkVariant=Disabled  SumVariant=Sum_PID  TsampFilterVariant=InternalTs  TsampNgainVariant=Passthrough  TsampIntegralVariant=Disabled_SignalSpec  ExternalSaturationOutDataTypeStr=Inherit: Same as second input  DerivativeSourceVariant=ErrorSignal
  Scope : Scope
  Sum : Sum  Inputs=|+-
  Ia ref* : Outport
  wires:
  PID Controller2/1 -> Scope/1, Ia ref*/1
  Divide/1 -> PID Controller2/1
  Ref speed/1 -> Sum/1
  Act speed/1 -> Sum/2
  Sum/1 -> Divide/2  "Error"
  Constant/1 -> Divide/1
